simulink library "BSC_lib"  (Simulink 7.4)
settings: Solver=FixedStepDiscrete  StartTime=0.0  StopTime=Inf  FixedStep=0.01  RelTol=1e-3
Description:
  | $Author:Zhao XiangRi$
  | $Date:2015/04/15$
  | $Revision:1.0$
settings Model: Creator=zhaoxiangri  LastModifiedBy=sunsijun

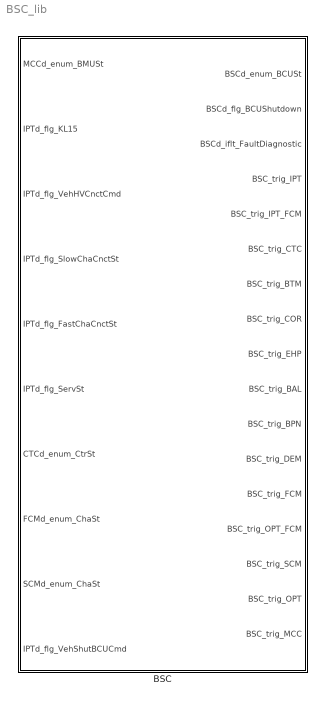
== system BSC_lib ==
  BSC : Subsystem  TreatAsAtomicUnit=on

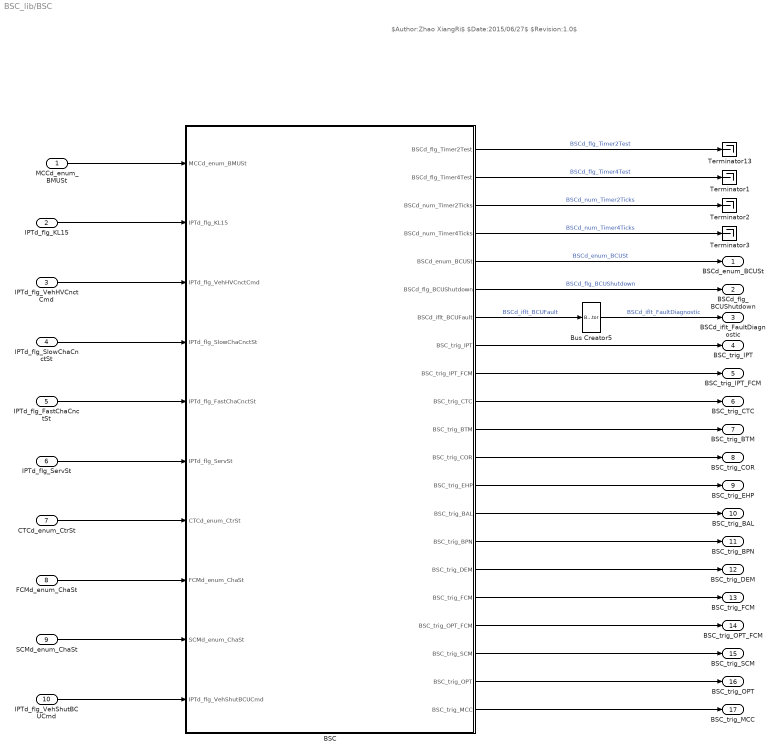
== system BSC_lib/BSC ==
  note: $Author:Zhao XiangRi$
      | $Date:2015/06/27$
      | $Revision:1.0$
  MCCd_enum_BMUSt : Inport  OutDataType=fixdt(1, 16)  OutScaling=2^0
  IPTd_flg_KL15 : Inport  Port=2  OutDataType=fixdt(1, 16)  OutScaling=2^0
  IPTd_flg_VehHVCnctCmd : Inport  Port=3  OutDataType=fixdt(1, 16)  OutScaling=2^0
  IPTd_flg_SlowChaCnctSt : Inport  Port=4  OutDataType=fixdt(1, 16)  OutScaling=2^0
  IPTd_flg_FastChaCnctSt : Inport  Port=5  OutDataType=fixdt(1, 16)  OutScaling=2^0
  IPTd_flg_ServSt : Inport  Port=6  OutDataType=fixdt(1, 16)  OutScaling=2^0
  CTCd_enum_CtrSt : Inport  Port=7  OutDataType=fixdt(1, 16)  OutScaling=2^0
  FCMd_enum_ChaSt : Inport  Port=8  OutDataType=fixdt(1, 16)  OutScaling=2^0
  SCMd_enum_ChaSt : Inport  Port=9  OutDataType=fixdt(1, 16)  OutScaling=2^0
  IPTd_flg_VehShutBCUCmd : Inport  Port=10  OutDataType=fixdt(1, 16)  OutScaling=2^0
  BSC : Stateflow chart  Description=|  TreatAsAtomicUnit=on
      | $Author:Zhao XiangRi$
      | $Date:2015/04/02$    
      | $Revision:1.0$
      settings: RTWFcnNameOpts=Use subsystem name  RTWFileNameOpts=Use function name
  Bus Creator5 : BusCreator  Inputs=1
  Terminator{1..3,13} (4 alike) : Terminator
  BSCd_enum_BCUSt : Outport  OutDataType=fixdt(1, 16)  OutScaling=2^0
  BSCd_flg_BCUShutdown : Outport  Port=2  OutDataType=fixdt(1, 16)  OutScaling=2^0
  BSCd_iflt_FaultDiagnostic : Outport  Port=3  OutDataType=fixdt(1, 16)  OutScaling=2^0
  BSC_trig_IPT : Outport  Port=4  OutDataType=fixdt(1, 16)  OutScaling=2^0
  BSC_trig_IPT_FCM : Outport  Port=5  OutDataType=fixdt(1, 16)  OutScaling=2^0
  BSC_trig_CTC : Outport  Port=6  OutDataType=fixdt(1, 16)  OutScaling=2^0
  BSC_trig_BTM : Outport  Port=7  OutDataType=fixdt(1, 16)  OutScaling=2^0
  BSC_trig_COR : Outport  Port=8  OutDataType=fixdt(1, 16)  OutScaling=2^0
  BSC_trig_EHP : Outport  Port=9  OutDataType=fixdt(1, 16)  OutScaling=2^0
  BSC_trig_BAL : Outport  Port=10  OutDataType=fixdt(1, 16)  OutScaling=2^0
  BSC_trig_BPN : Outport  Port=11  OutDataType=fixdt(1, 16)  OutScaling=2^0
  BSC_trig_DEM : Outport  Port=12  OutDataType=fixdt(1, 16)  OutScaling=2^0
  BSC_trig_FCM : Outport  Port=13  OutDataType=fixdt(1, 16)  OutScaling=2^0
  BSC_trig_OPT_FCM : Outport  Port=14  OutDataType=fixdt(1, 16)  OutScaling=2^0
  BSC_trig_SCM : Outport  Port=15  OutDataType=fixdt(1, 16)  OutScaling=2^0
  BSC_trig_OPT : Outport  Port=16  OutDataType=fixdt(1, 16)  OutScaling=2^0
  BSC_trig_MCC : Outport  Port=17  OutDataType=fixdt(1, 16)  OutScaling=2^0
  wires:
  BSC/4(BSCd_num_Timer4Ticks) -> Terminator3/1  "BSCd_num_Timer4Ticks"
  BSC/3(BSCd_num_Timer2Ticks) -> Terminator2/1  "BSCd_num_Timer2Ticks"
  BSC/2(BSCd_flg_Timer4Test) -> Terminator1/1  "BSCd_flg_Timer4Test"
  BSC/1(BSCd_flg_Timer2Test) -> Terminator13/1  "BSCd_flg_Timer2Test"
  BSC/18(BSC_trig_OPT_FCM) -> BSC_trig_OPT_FCM/1
  BSC/9(BSC_trig_IPT_FCM) -> BSC_trig_IPT_FCM/1
  SCMd_enum_ChaSt/1 -> BSC/9(SCMd_enum_ChaSt)
  BSC/7(BSCd_iflt_BCUFault) -> Bus Creator5/1  "BSCd_iflt_BCUFault"
  MCCd_enum_BMUSt/1 -> BSC/1(MCCd_enum_BMUSt)
  IPTd_flg_KL15/1 -> BSC/2(IPTd_flg_KL15)
  IPTd_flg_VehHVCnctCmd/1 -> BSC/3(IPTd_flg_VehHVCnctCmd)
  IPTd_flg_SlowChaCnctSt/1 -> BSC/4(IPTd_flg_SlowChaCnctSt)
  IPTd_flg_FastChaCnctSt/1 -> BSC/5(IPTd_flg_FastChaCnctSt)
  IPTd_flg_ServSt/1 -> BSC/6(IPTd_flg_ServSt)
  CTCd_enum_CtrSt/1 -> BSC/7(CTCd_enum_CtrSt)
  FCMd_enum_ChaSt/1 -> BSC/8(FCMd_enum_ChaSt)
  IPTd_flg_VehShutBCUCmd/1 -> BSC/10(IPTd_flg_VehShutBCUCmd)
  BSC/5(BSCd_enum_BCUSt) -> BSCd_enum_BCUSt/1  "BSCd_enum_BCUSt"
  BSC/6(BSCd_flg_BCUShutdown) -> BSCd_flg_BCUShutdown/1  "BSCd_flg_BCUShutdown"
  BSC/8(BSC_trig_IPT) -> BSC_trig_IPT/1
  BSC/10(BSC_trig_CTC) -> BSC_trig_CTC/1
  BSC/11(BSC_trig_BTM) -> BSC_trig_BTM/1
  BSC/12(BSC_trig_COR) -> BSC_trig_COR/1
  BSC/13(BSC_trig_EHP) -> BSC_trig_EHP/1
  BSC/14(BSC_trig_BAL) -> BSC_trig_BAL/1
  BSC/15(BSC_trig_BPN) -> BSC_trig_BPN/1
  BSC/16(BSC_trig_DEM) -> BSC_trig_DEM/1
  BSC/17(BSC_trig_FCM) -> BSC_trig_FCM/1
  BSC/19(BSC_trig_SCM) -> BSC_trig_SCM/1
  BSC/20(BSC_trig_OPT) -> BSC_trig_OPT/1
  BSC/21(BSC_trig_MCC) -> BSC_trig_MCC/1
  Bus Creator5/1 -> BSCd_iflt_FaultDiagnostic/1  "BSCd_iflt_FaultDiagnostic"

== stateflow chart BSC/BSC ==
  settings: description=|
      | $Author:Zhao XiangRi$
      | $Date:2015/03/26$
      | $Revision:1.0$
  state Selftest
    en:
    BSCd_enum_BCUSt=BCU_Selftest_St;
    BSCd_flg_BCUShutdown=0;
    BSCd_iflt_BCUFault=0;
    du:
    Timer.T1.Run(BSCc_tm_Selftest_max);
    BSC_trig_IPT;
    BSC_trig_MCC;
    BSC_trig_OPT;
    ex:
    Timer.T1.Clear();
  state Idle
    en:
    BSCd_enum_BCUSt=BCU_Idle_St;
    du:
    Timer.T2.Run(BSCc_tm_Idle_min);
    BSC_trig_IPT;
    BSC_trig_MCC;
    BSC_trig_COR;
    BSC_trig_EHP;
    BSC_trig_CTC;
    BSC_trig_BTM;
    BSC_trig_BPN;
    BSC_trig_DEM;
    BSC_trig_OPT;
    ex:
    Timer.T2.Clear();
  state Drive
    en:
    BSCd_enum_BCUSt=BCU_Drive_St ;
    du:
    BSC_trig_IPT;
    BSC_trig_MCC;
    BSC_trig_COR;
    BSC_trig_EHP;
    BSC_trig_CTC;
    BSC_trig_BTM;
    BSC_trig_BPN;
    BSC_trig_DEM;
    BSC_trig_OPT;
  state FastCharge
    en:
    BSCd_enum_BCUSt=BCU_FastCharge_St;
    du:
    BSC_trig_IPT;
    BSC_trig_IPT_FCM;
    BSC_trig_MCC;
    BSC_trig_COR;
    BSC_trig_EHP;
    BSC_trig_CTC;
    BSC_trig_BTM;
    BSC_trig_BPN;
    BSC_trig_DEM;
    BSC_trig_FCM;
    BSC_trig_BAL;
    BSC_trig_OPT;
    BSC_trig_OPT_FCM;
  state SlowCharge
    en:
    BSCd_enum_BCUSt=BCU_SlowCharge_St;
    du:
    BSC_trig_IPT;
    BSC_trig_MCC;
    BSC_trig_COR;
    BSC_trig_EHP;
    BSC_trig_CTC;
    BSC_trig_BTM;
    BSC_trig_BPN;
    BSC_trig_DEM;
    BSC_trig_SCM;
    BSC_trig_BAL;
    BSC_trig_OPT;
  state Shutdown
    BSCd_enum_BCUSt=BCU_Shutdown_St;
    BSCd_flg_BCUShutdown=1;
  state Powerlatch
    en:
    BSCd_enum_BCUSt=BCU_Powerlatch_St;
    du:
    Timer.T2.Run(BSCc_tm_PowerlatchWait);
    Timer.T4.Run(BSCc_tm_PowerlatchWait_max);
    BSC_trig_IPT;
    BSC_trig_MCC;
    BSC_trig_OPT;
    BSCd_flg_Timer4Test = Timer.T4.Timeout; %Added by Sun Sijun for test.
    BSCd_flg_Timer2Test = Timer.T2.Timeout;
    ex:
    Timer.T2.Clear();
    Timer.T4.Clear();
  state Service
    en:
    BSCd_enum_BCUSt=BCU_Service_St;
    du:
    BSC_trig_IPT;
    BSC_trig_CTC;
    BSC_trig_OPT;
  state Fault
    en:
    BSCd_enum_BCUSt=BCU_Fault_St;
    du:
    Timer.T3.Run(BSCc_tm_Fault_min);
    BSC_trig_IPT;
    BSC_trig_DEM;
    BSC_trig_OPT;
    BSCd_iflt_BCUFault=1;
    ex:
    Timer.T3.Clear();
  state Timer [function]
    settings: description=$Author:Zhao XiangRi$
    state T1 [function]
      settings: description=$Author:Zhao XiangRi$
      state Run(Limit) [function]
        settings: description=$Author:Zhao XiangRi$
        (default) -> (junction 25)
        (junction 25) -> (junction 26) [order 1] : [Init != 1]
            | {TimeTicks = 0;TimeLimit = Limit/10;Init = 1;}
        (junction 26) -> (junction 25)
        (junction 25) -> (junction 27) [order 2] : {TimeTicks++;}
        (junction 27) -> (junction 28) [order 1] : [TimeTicks >= TimeLimit]{Timeout = 1;}
        (junction 27) -> (junction 29) [order 2]
      state Clear [function]
        settings: description=$Author:Zhao XiangRi$
        (default) -> (junction 30)
        (junction 30) -> (junction 31) : {Timeout = 0;Init = 0;}
    state T2 [function]
      settings: description=$Author:Zhao XiangRi$
      state Run(Limit) [function]
        settings: description=$Author:Zhao XiangRi$
        (default) -> (junction 32)
        (junction 32) -> (junction 33) [order 1] : [Init != 1]{TimeTicks = 0;TimeLimit = Limit /10;Init = 1;}
        (junction 33) -> (junction 32)
        (junction 32) -> (junction 34) [order 2] : {TimeTicks++;
            | BSCd_num_Timer2Ticks=TimeTicks;}% Added by SSJ
        (junction 34) -> (junction 35) [order 1] : [TimeTicks >= TimeLimit]{Timeout = 1;}
        (junction 34) -> (junction 36) [order 2]
      state Clear [function]
        settings: description=$Author:Zhao XiangRi$
        (default) -> (junction 37)
        (junction 37) -> (junction 38) : {Timeout = 0;
            | Init = 0;}
    state T3 [function]
      settings: description=$Author:Zhao XiangRi$
      state Run(Limit) [function]
        settings: description=$Author:Zhao XiangRi$
        (default) -> (junction 39)
        (junction 39) -> (junction 40) [order 1] : [Init != 1]{TimeTicks = 0;TimeLimit = Limit/10;Init = 1;}
        (junction 40) -> (junction 39)
        (junction 39) -> (junction 41) [order 2] : {TimeTicks++;}
        (junction 41) -> (junction 42) [order 1] : [TimeTicks >= TimeLimit]{Timeout = 1;}
        (junction 41) -> (junction 43) [order 2]
      state Clear [function]
        settings: description=$Author:Zhao XiangRi$
        (default) -> (junction 44)
        (junction 44) -> (junction 45) : {Timeout = 0;Init = 0;}
    state T4 [function]
      settings: description=$Author:Zhao XiangRi$
      state Run(Limit) [function]
        settings: description=$Author:Zhao XiangRi$
        (default) -> (junction 46)
        (junction 46) -> (junction 47) [order 1] : [Init != 1]{TimeTicks = 0;TimeLimit = Limit/10 ;Init = 1;}
        (junction 47) -> (junction 46)
        (junction 46) -> (junction 48) [order 2] : {TimeTicks++;...
            | BSCd_num_Timer4Ticks=TimeTicks;}% Added by SSJ
        (junction 48) -> (junction 49) [order 1] : [TimeTicks >= TimeLimit]{Timeout = 1;}
        (junction 48) -> (junction 50) [order 2]
      state Clear [function]
        settings: description=$Author:Zhao XiangRi$
        (default) -> (junction 51)
        (junction 51) -> (junction 52) : {Timeout = 0;Init = 0;}
  Idle -> (junction 60) [order 3] : [IPTd_flg_SlowChaCnctSt==1&&...
      | IPTd_flg_FastChaCnctSt==0&&...
      | IPTd_flg_VehHVCnctCmd==0&&...
      | IPTd_flg_ServSt==0]
  Drive -> Powerlatch : [IPTd_flg_KL15==0&&...
      | CTCd_enum_CtrSt==CTC_DefaultOffline_St]
  Powerlatch -> (junction 57) [order 1] : [IPTd_flg_KL15==1||...
      | IPTd_flg_FastChaCnctSt==1||...
      | IPTd_flg_SlowChaCnctSt==1]
  Powerlatch -> Shutdown [order 2] : [MCCd_enum_BMUSt==BMU_Shutdown_St&&...
      | (IPTd_flg_VehShutBCUCmd==1||Timer.T2.Timeout==1)]
  FastCharge -> Powerlatch : [IPTd_flg_FastChaCnctSt==0&&...
      | CTCd_enum_CtrSt==CTC_DefaultOffline_St&&...
      | FCMd_enum_ChaSt==FCM_ChaFinished_St]
  Service -> (junction 63) : [IPTd_flg_ServSt==0&&...
      | CTCd_enum_CtrSt==CTC_DefaultOffline_St]
  Selftest -> (junction 59) [order 2] : [(Timer.T1.Timeout==1)&&(MCCd_enum_BMUSt!=BMU_Run_St)]
  Fault -> (junction 53) [order 1] : [Timer.T3.Timeout==1&&...
      | IPTd_flg_KL15==0&&...
      | IPTd_flg_FastChaCnctSt==0&&...
      | IPTd_flg_SlowChaCnctSt==0&&...
      | IPTd_flg_ServSt==0]
  Idle -> (junction 55) [order 2] : [Timer.T2.Timeout==1&&...
      | IPTd_flg_KL15==0&&...
      | IPTd_flg_FastChaCnctSt==0&&...
      | IPTd_flg_SlowChaCnctSt==0&&...
      | IPTd_flg_ServSt==0]
  Selftest -> Idle [order 1] : [MCCd_enum_BMUSt==BMU_Run_St]
  Idle -> Drive [order 4] : [IPTd_flg_VehHVCnctCmd==1&&...
      | IPTd_flg_FastChaCnctSt==0&&...
      | IPTd_flg_SlowChaCnctSt==0&&...
      | IPTd_flg_ServSt==0]
  Idle -> FastCharge [order 1] : [IPTd_flg_FastChaCnctSt==1&&...
      | IPTd_flg_VehHVCnctCmd==0&&...
      | IPTd_flg_SlowChaCnctSt==0&&...
      | IPTd_flg_ServSt==0]
  SlowCharge -> (junction 62) : [IPTd_flg_SlowChaCnctSt==0&&...
      | CTCd_enum_CtrSt==CTC_DefaultOffline_St&&...
      | SCMd_enum_ChaSt==SCM_NoCharge_St]
  Idle -> (junction 61) [order 5] : [IPTd_flg_ServSt==1&&...
      | IPTd_flg_FastChaCnctSt==0&&...
      | IPTd_flg_SlowChaCnctSt==0&&...
      | IPTd_flg_VehHVCnctCmd==0]
  (junction 64) -> Shutdown
  Idle -> Fault [order 6] : [(IPTd_flg_FastChaCnctSt==1&&IPTd_flg_SlowChaCnctSt==1)||...
      | (IPTd_flg_FastChaCnctSt==1&&IPTd_flg_VehHVCnctCmd==1)||...
      | (IPTd_flg_FastChaCnctSt==1&&IPTd_flg_ServSt==1)||...
      | (IPTd_flg_SlowChaCnctSt==1&&IPTd_flg_VehHVCnctCmd==1)||...
      | (IPTd_flg_SlowChaCnctSt==1&&IPTd_flg_ServSt==1)||...
      | (IPTd_flg_VehHVCnctCmd==1&&IPTd_flg_ServSt==1)]
  (default) -> Selftest
  (junction 54) -> (junction 64)
  (junction 53) -> (junction 54)
  (junction 56) -> Powerlatch
  (junction 55) -> (junction 56)
  (junction 57) -> (junction 58)
  (junction 58) -> Selftest
  (junction 59) -> Fault
  (junction 60) -> SlowCharge
  (junction 61) -> Service
  (junction 62) -> Powerlatch
  (junction 63) -> Powerlatch [order 1] : [IPTd_flg_KL15==1]
  (junction 63) -> (junction 64) [order 2] : [IPTd_flg_KL15==0]
  Powerlatch -> Shutdown [order 3] : [Timer.T4.Timeout==1]
  Fault -> Selftest [order 2] : [BSCc_flg_FaultTest]
  data: Timeout local boolean; TimeLimit local uint16; TimeTicks local uint16; Init local boolean; Limit function_input uint16; Timeout local boolean; TimeLimit local uint16; TimeTicks local uint16; Init local boolean; Limit function_input uint16; Timeout local boolean; TimeLimit local uint16; TimeTicks local uint16; Init local boolean; Limit function_input uint16; Timeout local boolean; TimeLimit local uint16; TimeTicks local uint16; Init local boolean; Limit function_input uint16; BSCd_flg_Timer2Test output boolean; BSCd_flg_Timer4Test output boolean; BSCd_num_Timer2Ticks output uint16; BSCd_num_Timer4Ticks output uint16; MCCd_enum_BMUSt input uint8; IPTd_flg_KL15 input boolean; IPTd_flg_VehHVCnctCmd input boolean; IPTd_flg_SlowChaCnctSt input boolean; IPTd_flg_FastChaCnctSt input boolean; IPTd_flg_ServSt input boolean; CTCd_enum_CtrSt input uint8; FCMd_enum_ChaSt input uint8; SCMd_enum_ChaSt input uint8; BSCd_enum_BCUSt output uint8; IPTd_flg_VehShutBCUCmd input boolean; BCU_FastCharge_St parameter uint8; BCU_Idle_St parameter uint8; BCU_Selftest_St parameter uint8; BCU_SlowCharge_St parameter uint8; BCU_Shutdown_St parameter uint8; BCU_Drive_St parameter uint8; BCU_Powerlatch_St parameter uint8; CTC_DriveOffline_St parameter uint8; BMU_Run_St parameter uint8; BCU_Service_St parameter uint8; BSCd_flg_BCUShutdown output boolean; BSCc_tm_Selftest_max parameter uint16; BMU_Shutdown_St parameter uint8; CTC_DefaultOffline_St parameter uint8; CTC_FastChaOffline_St parameter uint8; CTC_SlowChaOffline_St parameter uint8; BCU_Fault_St parameter uint8; CTC_ServiceOffline_St parameter uint8; SCM_NoCharge_St parameter uint8; FCM_ChaFinished_St parameter uint8; BSCd_iflt_BCUFault output boolean; BSCc_tm_PowerlatchWait parameter uint16; BSCc_tm_Idle_min parameter uint16; BSCc_tm_Fault_min parameter uint16; BSCc_tm_PowerlatchWait_max parameter uint16; BSCc_flg_FaultTest parameter boolean
  events: BSC_trig_IPT output FUNCTION_CALL_EVENT; BSC_trig_IPT_FCM output FUNCTION_CALL_EVENT; BSC_trig_CTC output FUNCTION_CALL_EVENT; BSC_trig_BTM output FUNCTION_CALL_EVENT; BSC_trig_COR output FUNCTION_CALL_EVENT; BSC_trig_EHP output FUNCTION_CALL_EVENT; BSC_trig_BAL output FUNCTION_CALL_EVENT; BSC_trig_BPN output FUNCTION_CALL_EVENT; BSC_trig_DEM output FUNCTION_CALL_EVENT; BSC_trig_FCM output FUNCTION_CALL_EVENT; BSC_trig_OPT_FCM output FUNCTION_CALL_EVENT; BSC_trig_SCM output FUNCTION_CALL_EVENT; BSC_trig_OPT output FUNCTION_CALL_EVENT; BSC_trig_MCC output FUNCTION_CALL_EVENT
